simulink model "breakingDownIntoComponents"  (R2025a)
settings: Solver=VariableStepAuto  StartTime=0.0  StopTime=10.0  RelTol=1e-3
libraries: SignalEditorBlockLib x1
settings Model: Creator=JPIRES3  LastModifiedBy=JPIRES3

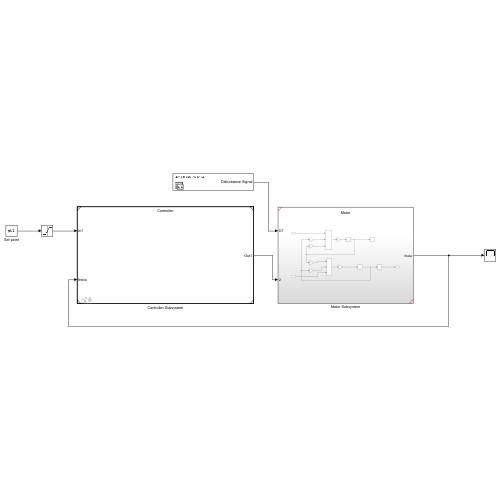
[thumbnail: Simulink's stored preview of the top-level diagram]
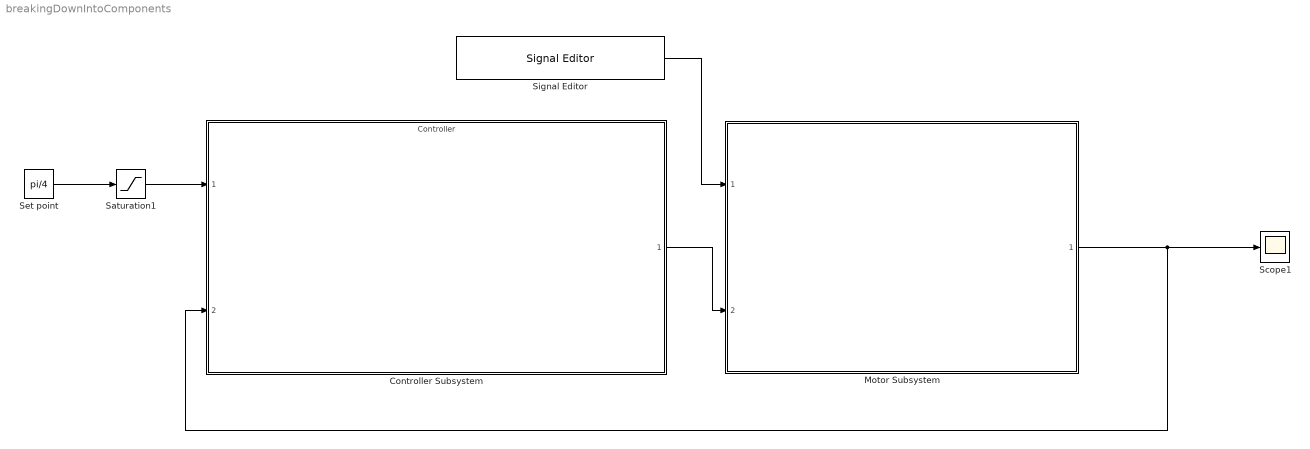
== system breakingDownIntoComponents ==
  Controller Subsystem : ModelReference  ModelNameDialog=Controller  UsingDefaultArgumentValue=0,0,0  SimulationMode=Normal  ModelReferenceVersion=1.3  Ts=0.01  ki=7.33  kp=9.39
  Motor Subsystem : Subsystem  ReferencedSubsystem=Motor
  Saturation1 : Saturate  UpperLimit=pi/4  LowerLimit=-pi/4
  Scope1 : Scope
      settings: ActiveDisplayYMinimum=-0.11554258584712604  ActiveDisplayYMaximum=1.0398832726241345
  Set point : Constant  Value=pi/4
  Signal Editor : SignalEditorBlockLib/Signal Editor  FileName=C:\Users\jpires3\Documents\Matlab-projects\Module 3 - Introduction to subsystems\Disturbance.mat  ActiveScenario=SmallDisturbance  ActiveSignal=Disturbance Signal  IsBus=off  OutputBusObjectStr=Bus: BusObject  SampleTime=0  ZeroCross=off  OutputAfterFinalValue=Setting to zero  Unit=inherit  PreserveSignalName=on  ApplySigPropsToAllScenarios=on  ApplySigPropsToAllSignals=off  SignalPropertySource=Dialog parameters
  wires:
  Set point/1 -> Saturation1/1
  Signal Editor/1 -> Motor Subsystem/1
  Controller Subsystem/1 -> Motor Subsystem/2
  Saturation1/1 -> Controller Subsystem/1
  Motor Subsystem/1 -> Controller Subsystem/2, Scope1/1
